simulink model "first_project"  (R2020a)
settings: Solver=VariableStepAuto  StartTime=0.0  StopTime=10.0  RelTol=1e-3
settings Model: Creator=mluser  LastModifiedBy=mluser

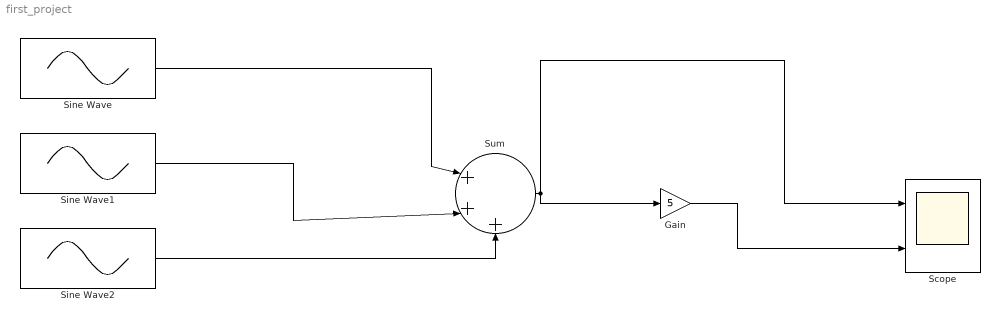
== system first_project ==
  Gain : Gain  Gain=5
  Scope : Scope  NumInputPorts=2
  Sine Wave : Sin  SampleTime=0
  Sine Wave1 : Sin  Amplitude=5  SampleTime=0
  Sine Wave2 : Sin  Amplitude=10  SampleTime=0
  Sum : Sum  Inputs=|+++
  wires:
  Sine Wave/1 -> Sum/1
  Sine Wave1/1 -> Sum/2
  Sine Wave2/1 -> Sum/3
  Sum/1 -> Gain/1, Scope/1
  Gain/1 -> Scope/2
